simulink model "Motor_Fault_Detection_System"  (R2025b)
settings: Solver=ode4  StartTime=0.0  StopTime=10  FixedStep=0.01  RelTol=1e-3
undefined symbols (not defined in the file or in its folder): magnitude
settings Model: Creator=anifa  LastModifiedBy=anifa

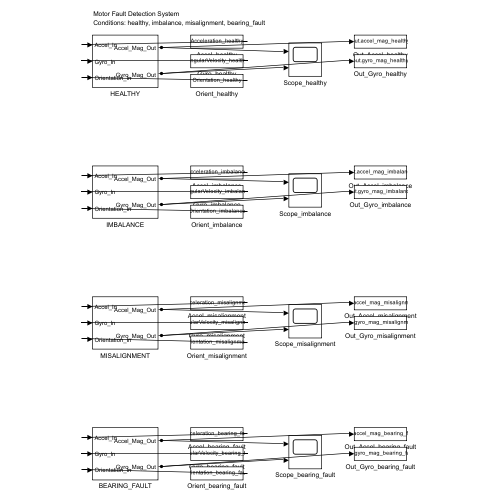
[thumbnail: Simulink's stored preview of the top-level diagram]
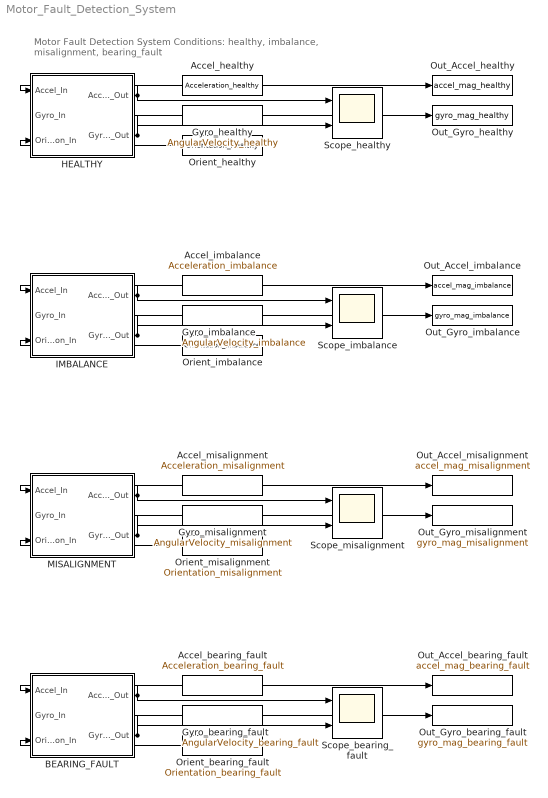
== system Motor_Fault_Detection_System ==
  note: Motor Fault Detection System
      | Conditions: healthy, imbalance, misalignment, bearing_fault
  Accel_bearing_fault : FromWorkspace  VariableName=Acceleration_bearing_fault
  Accel_healthy : FromWorkspace  VariableName=Acceleration_healthy
  Accel_imbalance : FromWorkspace  VariableName=Acceleration_imbalance
  Accel_misalignment : FromWorkspace  VariableName=Acceleration_misalignment
  BEARING_FAULT : Subsystem
  Gyro_bearing_fault : FromWorkspace  VariableName=AngularVelocity_bearing_fault
  Gyro_healthy : FromWorkspace  VariableName=AngularVelocity_healthy
  Gyro_imbalance : FromWorkspace  VariableName=AngularVelocity_imbalance
  Gyro_misalignment : FromWorkspace  VariableName=AngularVelocity_misalignment
  HEALTHY : Subsystem
  IMBALANCE : Subsystem
  MISALIGNMENT : Subsystem
  Orient_bearing_fault : FromWorkspace  VariableName=Orientation_bearing_fault
  Orient_healthy : FromWorkspace  VariableName=Orientation_healthy
  Orient_imbalance : FromWorkspace  VariableName=Orientation_imbalance
  Orient_misalignment : FromWorkspace  VariableName=Orientation_misalignment
  Out_Accel_bearing_fault : ToWorkspace  VariableName=accel_mag_bearing_fault  SaveFormat=Timeseries  SampleTime=-1
  Out_Accel_healthy : ToWorkspace  VariableName=accel_mag_healthy  SaveFormat=Timeseries  SampleTime=-1
  Out_Accel_imbalance : ToWorkspace  VariableName=accel_mag_imbalance  SaveFormat=Timeseries  SampleTime=-1
  Out_Accel_misalignment : ToWorkspace  VariableName=accel_mag_misalignment  SaveFormat=Timeseries  SampleTime=-1
  Out_Gyro_bearing_fault : ToWorkspace  VariableName=gyro_mag_bearing_fault  SaveFormat=Timeseries  SampleTime=-1
  Out_Gyro_healthy : ToWorkspace  VariableName=gyro_mag_healthy  SaveFormat=Timeseries  SampleTime=-1
  Out_Gyro_imbalance : ToWorkspace  VariableName=gyro_mag_imbalance  SaveFormat=Timeseries  SampleTime=-1
  Out_Gyro_misalignment : ToWorkspace  VariableName=gyro_mag_misalignment  SaveFormat=Timeseries  SampleTime=-1
  Scope_bearing_fault : Scope  NumInputPorts=2
  Scope_healthy : Scope  NumInputPorts=2
  Scope_imbalance : Scope  NumInputPorts=2
  Scope_misalignment : Scope  NumInputPorts=2
  wires:
  Accel_healthy/1 -> HEALTHY/1(Accel_In)
  Gyro_healthy/1 -> HEALTHY/2(Gyro_In)
  Orient_healthy/1 -> HEALTHY/3(Orientation_In)
  HEALTHY/1(Accel_Mag_Out) -> Scope_healthy/1, Out_Accel_healthy/1
  HEALTHY/2(Gyro_Mag_Out) -> Scope_healthy/2, Out_Gyro_healthy/1
  Accel_imbalance/1 -> IMBALANCE/1(Accel_In)
  Gyro_imbalance/1 -> IMBALANCE/2(Gyro_In)
  Orient_imbalance/1 -> IMBALANCE/3(Orientation_In)
  IMBALANCE/1(Accel_Mag_Out) -> Scope_imbalance/1, Out_Accel_imbalance/1
  IMBALANCE/2(Gyro_Mag_Out) -> Scope_imbalance/2, Out_Gyro_imbalance/1
  Accel_misalignment/1 -> MISALIGNMENT/1(Accel_In)
  Gyro_misalignment/1 -> MISALIGNMENT/2(Gyro_In)
  Orient_misalignment/1 -> MISALIGNMENT/3(Orientation_In)
  MISALIGNMENT/1(Accel_Mag_Out) -> Scope_misalignment/1, Out_Accel_misalignment/1
  MISALIGNMENT/2(Gyro_Mag_Out) -> Scope_misalignment/2, Out_Gyro_misalignment/1
  Accel_bearing_fault/1 -> BEARING_FAULT/1(Accel_In)
  Gyro_bearing_fault/1 -> BEARING_FAULT/2(Gyro_In)
  Orient_bearing_fault/1 -> BEARING_FAULT/3(Orientation_In)
  BEARING_FAULT/1(Accel_Mag_Out) -> Scope_bearing_fault/1, Out_Accel_bearing_fault/1
  BEARING_FAULT/2(Gyro_Mag_Out) -> Scope_bearing_fault/2, Out_Gyro_bearing_fault/1

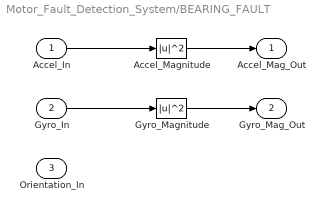
== system Motor_Fault_Detection_System/BEARING_FAULT ==
  Accel_In : Inport
  Gyro_In : Inport  Port=2
  Orientation_In : Inport  Port=3
  Accel_Magnitude : Math  Operator=magnitude^2
  Gyro_Magnitude : Math  Operator=magnitude^2
  Accel_Mag_Out : Outport
  Gyro_Mag_Out : Outport  Port=2
  wires:
  Accel_In/1 -> Accel_Magnitude/1
  Gyro_In/1 -> Gyro_Magnitude/1
  Accel_Magnitude/1 -> Accel_Mag_Out/1
  Gyro_Magnitude/1 -> Gyro_Mag_Out/1

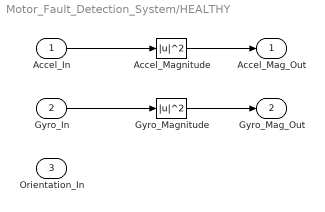
== system Motor_Fault_Detection_System/HEALTHY ==
  Accel_In : Inport
  Gyro_In : Inport  Port=2
  Orientation_In : Inport  Port=3
  Accel_Magnitude : Math  Operator=magnitude^2
  Gyro_Magnitude : Math  Operator=magnitude^2
  Accel_Mag_Out : Outport
  Gyro_Mag_Out : Outport  Port=2
  wires:
  Accel_In/1 -> Accel_Magnitude/1
  Gyro_In/1 -> Gyro_Magnitude/1
  Accel_Magnitude/1 -> Accel_Mag_Out/1
  Gyro_Magnitude/1 -> Gyro_Mag_Out/1

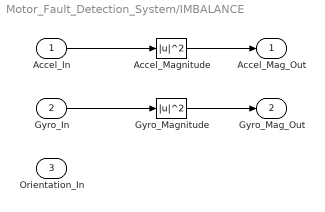
== system Motor_Fault_Detection_System/IMBALANCE ==
  Accel_In : Inport
  Gyro_In : Inport  Port=2
  Orientation_In : Inport  Port=3
  Accel_Magnitude : Math  Operator=magnitude^2
  Gyro_Magnitude : Math  Operator=magnitude^2
  Accel_Mag_Out : Outport
  Gyro_Mag_Out : Outport  Port=2
  wires:
  Accel_In/1 -> Accel_Magnitude/1
  Gyro_In/1 -> Gyro_Magnitude/1
  Accel_Magnitude/1 -> Accel_Mag_Out/1
  Gyro_Magnitude/1 -> Gyro_Mag_Out/1

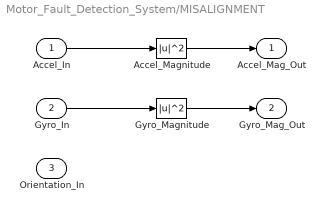
== system Motor_Fault_Detection_System/MISALIGNMENT ==
  Accel_In : Inport
  Gyro_In : Inport  Port=2
  Orientation_In : Inport  Port=3
  Accel_Magnitude : Math  Operator=magnitude^2
  Gyro_Magnitude : Math  Operator=magnitude^2
  Accel_Mag_Out : Outport
  Gyro_Mag_Out : Outport  Port=2
  wires:
  Accel_In/1 -> Accel_Magnitude/1
  Gyro_In/1 -> Gyro_Magnitude/1
  Accel_Magnitude/1 -> Accel_Mag_Out/1
  Gyro_Magnitude/1 -> Gyro_Mag_Out/1
